simulink model "MCU_vectorControl_dsPIC33AK128MC106_MCLV_48V_300W"  (R2024a)
settings: Solver=FixedStepDiscrete  StartTime=0.0  StopTime=10.0  FixedStep=50e-6  RelTol=1e-3  EnableMultiTasking=on
undefined symbols (not defined in the file or in its folder): A0, A4, ADC, B0, Bias1, Bias2, C10, C11, C6, C7, C8, control, D11, D12, DiscIntNeverNeededParam, inverter, Max, MaxPer, model, ms, NumBits1, NumBits2, P1, P17, P20, P39, P40, P41, P43, P44, P60, P61, Pin, PosRange1, PosRange2, PWM1_Trg1, Resol, s, Slope1, Slope2, us
libraries: simulink x43, MCHP_Blockset x23
(part 5 of 5)

== system MCU_vectorControl_dsPIC33AK128MC106_MCLV_48V_300W/BOARD MCLV-48V-300W dsPIC33AK128MC106 MC DIM/Downsample x20 ==
  note: DownSample & Average by changing data scaling
  In1 : Inport
  Compare To Constant : simulink/Logic and Bit Operations/Compare To Constant  relop===  const=1  OutDataTypeStr=boolean
  Counter Limited : simulink/Sources/Counter Limited  uplimit=DownSample-1  tsamp=-1
  Data Type Duplicate : DataTypeDuplicate
  Data Type Propagation : simulink/Signal Attributes/Data Type Propagation  PropDataType=fixdt(1, 16)  IfRefDouble=double  IfRefSingle=single  IsSigned=IsSigned1 or IsSigned2  NumBitsBase=NumBits1+NumBits2  NumBitsMult=1  NumBitsAdd=0  NumBitsAllowFinal=1:128  PropScaling=2^-10  ValuesUsedBestPrec=[5 -7]  SlopeBase=Slope1  SlopeMult=1  SlopeAdd=0  BiasBase=Bias1  BiasMult=1  BiasAdd=0
  Data Type Propagation1 : simulink/Signal Attributes/Data Type Propagation  PropDataType=fixdt(1, 16)  IfRefDouble=double  IfRefSingle=single  IsSigned=IsSigned1 or IsSigned2  NumBitsBase=NumBits1+NumBits2  NumBitsMult=1  NumBitsAdd=0  NumBitsAllowFinal=1:128  PropScaling=2^-10  ValuesUsedBestPrec=[5 -7]  SlopeBase=PosRange1  SlopeMult=1  SlopeAdd=0  BiasBase=Bias1  BiasMult=1  BiasAdd=0
  Discrete-Time Integrator : DiscreteIntegrator  IntegratorMethod=Accumulation: Backward Euler  gainval=1  ExternalReset=sampled level  SampleTime=-1  OutDataTypeStr=Inherit: Inherit via back propagation  ICPrevOutput=DiscIntNeverNeededParam  ICPrevScaledInput=DiscIntNeverNeededParam
  Gain : Gain  Gain=1/DownSample  OutDataTypeStr=Inherit: Inherit via back propagation  RndMeth=Round
  Gain1 : Gain  Gain=1/DownSample  OutDataTypeStr=Inherit: Inherit via back propagation
  Rate Transition1 : RateTransition  OutPortSampleTimeOpt=Multiple of input port sample time  OutPortSampleTimeMultiple=DownSample  OutPortSampleTime=DownSample
  Rate Transition3 : RateTransition  OutPortSampleTimeOpt=Multiple of input port sample time  OutPortSampleTimeMultiple=DownSample  OutPortSampleTime=DownSample
  Terminator : Terminator
  Out1 : Outport  VectorParamsAs1DForOutWhenUnconnected=off
  wires:
  Gain1/1 -> Data Type Propagation1/3, Terminator/1
  Rate Transition1/1 -> Data Type Duplicate/1, Data Type Propagation1/1, Data Type Propagation1/2
  Gain/1 -> Out1/1, Data Type Duplicate/2
  Counter Limited/1 -> Compare To Constant/1
  Discrete-Time Integrator/1 -> Rate Transition3/1, Data Type Propagation/3
  Compare To Constant/1 -> Discrete-Time Integrator/2
  In1/1 -> Data Type Propagation/1, Data Type Propagation/2, Discrete-Time Integrator/1, Rate Transition1/1
  Rate Transition3/1 -> Gain/1, Gain1/1

== system MCU_vectorControl_dsPIC33AK128MC106_MCLV_48V_300W/BOARD MCLV-48V-300W dsPIC33AK128MC106 MC DIM/Downsample x20 _ ==
  note: DownSample & Average by changing data scaling
  In1 : Inport
  Compare To Constant : simulink/Logic and Bit Operations/Compare To Constant  relop===  const=1  OutDataTypeStr=boolean
  Counter Limited : simulink/Sources/Counter Limited  uplimit=DownSample-1  tsamp=-1
  Data Type Duplicate : DataTypeDuplicate
  Data Type Propagation : simulink/Signal Attributes/Data Type Propagation  PropDataType=fixdt(1, 16)  IfRefDouble=double  IfRefSingle=single  IsSigned=IsSigned1 or IsSigned2  NumBitsBase=NumBits1+NumBits2  NumBitsMult=1  NumBitsAdd=0  NumBitsAllowFinal=1:128  PropScaling=2^-10  ValuesUsedBestPrec=[5 -7]  SlopeBase=Slope1  SlopeMult=1  SlopeAdd=0  BiasBase=Bias1  BiasMult=1  BiasAdd=0
  Data Type Propagation1 : simulink/Signal Attributes/Data Type Propagation  PropDataType=fixdt(1, 16)  IfRefDouble=double  IfRefSingle=single  IsSigned=IsSigned1 or IsSigned2  NumBitsBase=NumBits1+NumBits2  NumBitsMult=1  NumBitsAdd=0  NumBitsAllowFinal=1:128  PropScaling=2^-10  ValuesUsedBestPrec=[5 -7]  SlopeBase=PosRange1  SlopeMult=1  SlopeAdd=0  BiasBase=Bias1  BiasMult=1  BiasAdd=0
  Discrete-Time Integrator : DiscreteIntegrator  IntegratorMethod=Accumulation: Backward Euler  gainval=1  ExternalReset=sampled level  SampleTime=-1  OutDataTypeStr=Inherit: Inherit via back propagation  ICPrevOutput=DiscIntNeverNeededParam  ICPrevScaledInput=DiscIntNeverNeededParam
  Gain : Gain  Gain=1/DownSample  OutDataTypeStr=Inherit: Inherit via back propagation  RndMeth=Round
  Gain1 : Gain  Gain=1/DownSample  OutDataTypeStr=Inherit: Inherit via back propagation
  Rate Transition1 : RateTransition  OutPortSampleTimeOpt=Multiple of input port sample time  OutPortSampleTimeMultiple=DownSample  OutPortSampleTime=DownSample
  Rate Transition3 : RateTransition  OutPortSampleTimeOpt=Multiple of input port sample time  OutPortSampleTimeMultiple=DownSample  OutPortSampleTime=DownSample
  Terminator : Terminator
  Out1 : Outport  VectorParamsAs1DForOutWhenUnconnected=off
  wires:
  Rate Transition3/1 -> Gain1/1, Gain/1
  In1/1 -> Rate Transition1/1, Discrete-Time Integrator/1, Data Type Propagation/2, Data Type Propagation/1
  Compare To Constant/1 -> Discrete-Time Integrator/2
  Discrete-Time Integrator/1 -> Data Type Propagation/3, Rate Transition3/1
  Counter Limited/1 -> Compare To Constant/1
  Gain/1 -> Data Type Duplicate/2, Out1/1
  Rate Transition1/1 -> Data Type Propagation1/2, Data Type Propagation1/1, Data Type Duplicate/1
  Gain1/1 -> Terminator/1, Data Type Propagation1/3

== system MCU_vectorControl_dsPIC33AK128MC106_MCLV_48V_300W/BOARD MCLV-48V-300W dsPIC33AK128MC106 MC DIM/MCLV 48V-300W board webpage ==

== system MCU_vectorControl_dsPIC33AK128MC106_MCLV_48V_300W/BOARD MCLV-48V-300W dsPIC33AK128MC106 MC DIM/Timing Analysis ==
  note: CPU overload is 0 if no overload took place between two MCU Overload block execution.
      | Otherwise, bits field output code for TID(s) responsible for at least one overload.
  Downsample Averaged2 : Subsystem  mask{InputSampleTime=.001, DownSample=100}
      mask prompts: InputSampleTime "Input sample time"; DownSample "DownSample Factor"
  Gain : Gain  Gain=5e-9/.001 * 100  OutMin=0  OutMax=100  OutDataTypeStr=fixdt(0,16)  RndMeth=Simplest  SaturateOnIntegerOverflow=on
  MCU Load : MCHP_Blockset/Profiling/MCU Load  MCULoadPin_TXT=None  MCULoadMeasure=on  TIMER_Resolution_TXT="Resol: 0.005(us)  -  Max: 0.328(ms)"  MCHP_TIMER_REQUEST={MCU_Load}{MCU_Load}21:5:0:0:[]:32768;  MCHP_TIMER_RESULT=[2 65535 ]  MCHP_MASTERLINK=MCU_vectorControl_dsPIC33AK128MC106_MCLV_48V_300W/BOARD MCLV-48V-300W dsPIC33AK128MC106 MC DIM/Microchip Master  MCHP_COMPILED_INFO="CompiledSampleTime= [0.0010000000000000000208   0 ];CompiledInportDataTypes=[    ];CompiledInportDataWidth=[];"  Info="Timer 2:  Resol: 5(ns)  -  Max: 327.68(us)"  SampleTime=.001
      settings: SourceProductName=MPLAB Device Blocks for Simulink
  MCU Overload : MCHP_Blockset/Profiling/MCU Overload  MCUOverloadBlockOutput=on  MCUOverLoadPin_TXT=None  MCHP_MASTERLINK=MCU_vectorControl_dsPIC33AK128MC106_MCLV_48V_300W/BOARD MCLV-48V-300W dsPIC33AK128MC106 MC DIM/Microchip Master  SampleTime=-1
      settings: SourceProductName=MPLAB Device Blocks for Simulink
  Overload : Constant  Value=65535  OutDataTypeStr=Inherit: Inherit via back propagation
  Rate Transition : RateTransition  Deterministic=off  OutPortSampleTime=.0005*200
  Switch : Switch  Criteria=u2 ~= 0  SaturateOnIntegerOverflow=off  InputSameDT=off
  CPU Load : Outport  Unit=%  SampleTime=.0005*200
  CPU Overload : Outport  Port=2
  wires:
  Gain/1 -> CPU Load/1
  Overload/1 -> Switch/1
  Switch/1 -> Gain/1
  Downsample Averaged2/1(Out1) -> Switch/3
  MCU Load/1 -> Downsample Averaged2/1(In1)
  MCU Overload/1 -> CPU Overload/1, Rate Transition/1
  Rate Transition/1 -> Switch/2

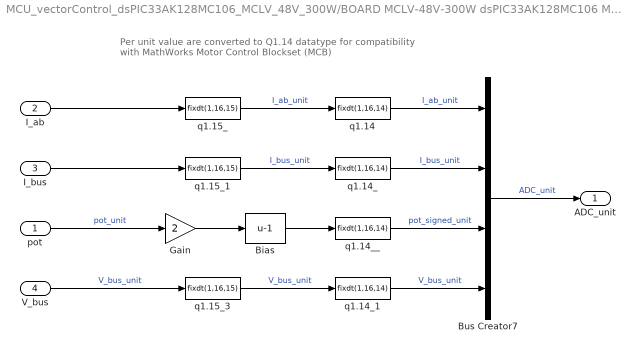
== system MCU_vectorControl_dsPIC33AK128MC106_MCLV_48V_300W/BOARD MCLV-48V-300W dsPIC33AK128MC106 MC DIM/per_unit ==
  note: Per unit value are converted to Q1.14 datatype
      | for compatibility with MathWorks Motor Control Blockset (MCB)
  pot : Inport
  I_ab : Inport  Port=2
  I_bus : Inport  Port=3
  V_bus : Inport  Port=4
  Bias : Bias  Bias=-1  SaturateOnIntegerOverflow=off
  Bus Creator7 : BusCreator  Inputs=4
  Gain : Gain  Gain=2  OutDataTypeStr=fixdt(1,16,15)  LockScale=on
  q1.14 : DataTypeConversion  OutDataTypeStr=fixdt(1,16,14)  SaturateOnIntegerOverflow=off  RndMeth=Floor  LockScale=on
  q1.14_ : DataTypeConversion  OutDataTypeStr=fixdt(1,16,14)  SaturateOnIntegerOverflow=off  RndMeth=Floor  LockScale=on
  q1.14_1 : DataTypeConversion  OutDataTypeStr=fixdt(1,16,14)  SaturateOnIntegerOverflow=off  RndMeth=Floor  LockScale=on
  q1.14__ : DataTypeConversion  OutDataTypeStr=fixdt(1,16,14)  SaturateOnIntegerOverflow=off  RndMeth=Floor  LockScale=on
  q1.15_ : DataTypeConversion  OutDataTypeStr=fixdt(1,16,15)  ConvertRealWorld=Stored Integer (SI)  SaturateOnIntegerOverflow=off  RndMeth=Floor  LockScale=on
  q1.15_1 : DataTypeConversion  OutDataTypeStr=fixdt(1,16,15)  ConvertRealWorld=Stored Integer (SI)  SaturateOnIntegerOverflow=off  RndMeth=Floor  LockScale=on
  q1.15_3 : DataTypeConversion  OutDataTypeStr=fixdt(1,16,15)  ConvertRealWorld=Stored Integer (SI)  SaturateOnIntegerOverflow=off  RndMeth=Floor  LockScale=on
  ADC_unit : Outport
  wires:
  Bias/1 -> q1.14__/1
  Gain/1 -> Bias/1
  q1.14_1/1 -> Bus Creator7/4  "V_bus_unit"
  q1.14__/1 -> Bus Creator7/3  "pot_signed_unit"
  q1.14_/1 -> Bus Creator7/2  "I_bus_unit"
  q1.14/1 -> Bus Creator7/1  "I_ab_unit"
  q1.15_3/1 -> q1.14_1/1  "V_bus_unit"
  Bus Creator7/1 -> ADC_unit/1  "ADC_unit"
  q1.15_/1 -> q1.14/1  "I_ab_unit"
  q1.15_1/1 -> q1.14_/1  "I_bus_unit"
  I_bus/1 -> q1.15_1/1
  pot/1 -> Gain/1  "pot_unit"
  V_bus/1 -> q1.15_3/1  "V_bus_unit"
  I_ab/1 -> q1.15_/1

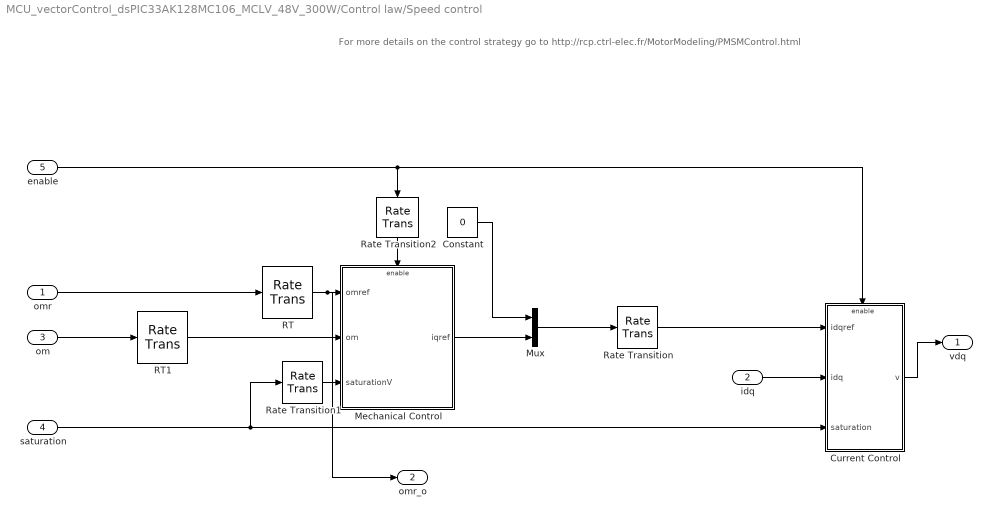
== system MCU_vectorControl_dsPIC33AK128MC106_MCLV_48V_300W/Control law/Speed control ==
  note: For more details on the control strategy go to
      |
      | http://rcp.ctrl-elec.fr/MotorModeling/PMSMControl.html
  omr : Inport
  idq : Inport  Port=2
  om : Inport  Port=3
  saturation : Inport  Port=4
  enable : Inport  Port=5
  Constant : Constant  Value=0  OutDataTypeStr=Inherit: Inherit via back propagation
  Current Control : Subsystem
  Mechanical Control : Subsystem
  Mux : Mux  Inputs=2
  RT : RateTransition  OutPortSampleTime=0.001
  RT1 : RateTransition  OutPortSampleTime=0.001
  Rate Transition : RateTransition
  Rate Transition1 : RateTransition  OutPortSampleTime=control.tsMeca
  Rate Transition2 : RateTransition
  vdq : Outport
  omr_o : Outport  Port=2
  wires:
  RT1/1 -> Mechanical Control/2(om)
  RT/1 -> omr_o/1, Mechanical Control/1(omref)
  idq/1 -> Current Control/2(idq)
  Mux/1 -> Rate Transition/1
  Current Control/1(v) -> vdq/1
  saturation/1 -> Rate Transition1/1, Current Control/3(saturation)
  om/1 -> RT1/1
  Constant/1 -> Mux/1
  Mechanical Control/1(iqref) -> Mux/2
  Rate Transition/1 -> Current Control/1(idqref)
  omr/1 -> RT/1
  Rate Transition1/1 -> Mechanical Control/3(saturationV)
  enable/1 -> Current Control/Enable, Rate Transition2/1
  Rate Transition2/1 -> Mechanical Control/Enable

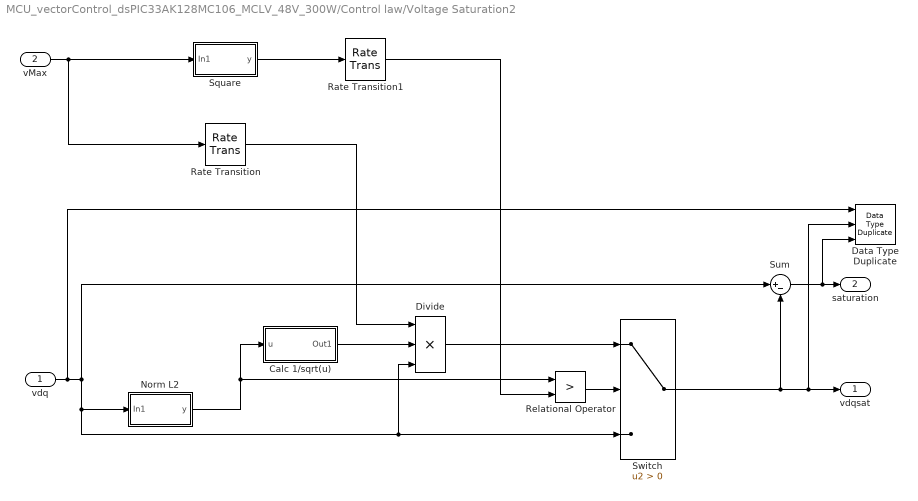
== system MCU_vectorControl_dsPIC33AK128MC106_MCLV_48V_300W/Control law/Voltage Saturation2 ==
  vdq : Inport
  vMax : Inport  Port=2
  Calc 1/sqrt(u) : Subsystem
  Data Type Duplicate : DataTypeDuplicate  NumInputPorts=3
  Divide : Product  Inputs=***  OutDataTypeStr=Inherit: Inherit via back propagation  SaturateOnIntegerOverflow=on
  Norm L2 : Subsystem
  Rate Transition : RateTransition
  Rate Transition1 : RateTransition
  Relational Operator : RelationalOperator  Operator=>  OutDataTypeStr=boolean  RndMeth=Simplest  InputSameDT=off
  Square : Subsystem
  Sum : Sum  Inputs=|+-  OutDataTypeStr=Inherit: Inherit via back propagation  SaturateOnIntegerOverflow=on
  Switch : Switch  Criteria=u2 > Threshold  OutDataTypeStr=Inherit: Inherit via back propagation  SaturateOnIntegerOverflow=off  InputSameDT=off
  vdqsat : Outport  VectorParamsAs1DForOutWhenUnconnected=off
  saturation : Outport  Port=2  VectorParamsAs1DForOutWhenUnconnected=off
  wires:
  Divide/1 -> Switch/1
  Norm L2/1(y) -> Calc 1/sqrt(u)/1(u), Relational Operator/1
  Switch/1 -> vdqsat/1, Data Type Duplicate/2, Sum/2
  vdq/1 -> Sum/1, Switch/3, Divide/3, Norm L2/1(In1), Data Type Duplicate/1
  Sum/1 -> saturation/1, Data Type Duplicate/3
  Relational Operator/1 -> Switch/2
  vMax/1 -> Square/1(In1), Rate Transition/1
  Square/1(y) -> Rate Transition1/1
  Rate Transition/1 -> Divide/1
  Rate Transition1/1 -> Relational Operator/2
  Calc 1/sqrt(u)/1(Out1) -> Divide/2

== system MCU_vectorControl_dsPIC33AK128MC106_MCLV_48V_300W/Control law/off1 ==
  Mux : Mux  Inputs=2
  vd : Constant  Value=0  OutDataTypeStr=Inherit: Inherit via back propagation
  vq : Constant  Value=0  OutDataTypeStr=Inherit: Inherit via back propagation
  vdq : Outport  VectorParamsAs1DForOutWhenUnconnected=off
  wires:
  vd/1 -> Mux/1
  Mux/1 -> vdq/1
  vq/1 -> Mux/2

== system MCU_vectorControl_dsPIC33AK128MC106_MCLV_48V_300W/Control law/open loop ==
  vdqr : Inport
  Enable : EnablePort
  vdq : Outport  VectorParamsAs1DForOutWhenUnconnected=off
  wires:
  vdqr/1 -> vdq/1

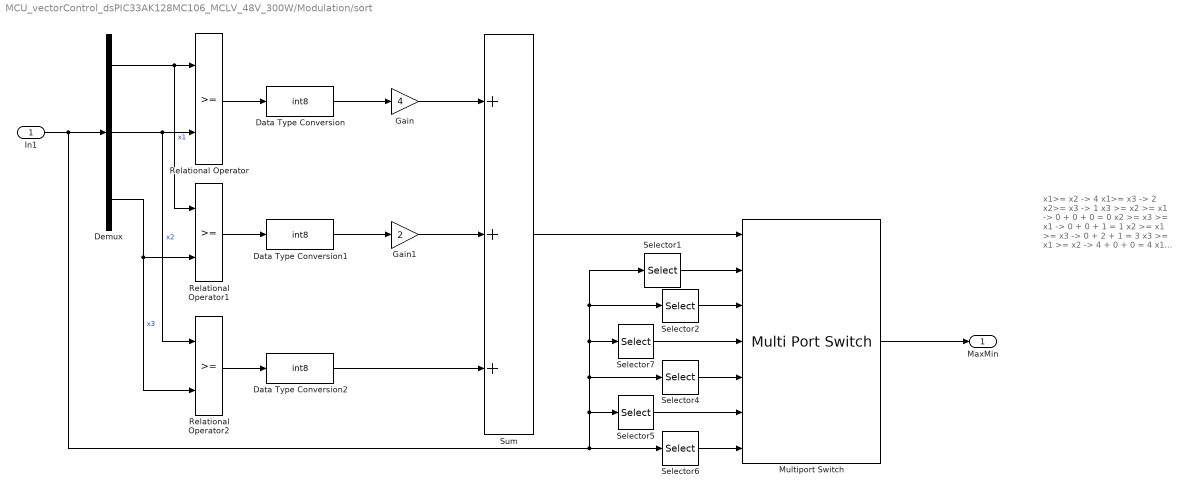
== system MCU_vectorControl_dsPIC33AK128MC106_MCLV_48V_300W/Modulation/sort ==
  note: x1>= x2 -> 4
      | x1>= x3 -> 2
      | x2>= x3 -> 1
      |
      | x3 >= x2 >= x1 -> 0 + 0 + 0 = 0
      | x2 >= x3 >= x1 -> 0 + 0 + 1 = 1
      | x2 >= x1 >= x3 -> 0 + 2 + 1 = 3
      | x3 >= x1 >= x2 -> 4 + 0 + 0 = 4
      | x1 >= x3 >= x2 -> 4 + 2 + 0 = 6
      | x1 >= x2 >= x3 -> 4 + 2 + 1 = 7
  In1 : Inport
  Data Type Conversion : DataTypeConversion  OutDataTypeStr=int8  SaturateOnIntegerOverflow=off  RndMeth=Floor
  Data Type Conversion1 : DataTypeConversion  OutDataTypeStr=int8  SaturateOnIntegerOverflow=off  RndMeth=Floor
  Data Type Conversion2 : DataTypeConversion  OutDataTypeStr=int8  SaturateOnIntegerOverflow=off  RndMeth=Floor
  Demux : Demux  Outputs=3
  Gain : Gain  Gain=4  OutDataTypeStr=Inherit: Same as input
  Gain1 : Gain  Gain=2  OutDataTypeStr=Inherit: Same as input
  Multiport Switch : MultiPortSwitch  DataPortOrder=Specify indices  DataPortIndices={0,1,3,4,6,7}  SaturateOnIntegerOverflow=off  InputSameDT=off
  Relational Operator : RelationalOperator  OutDataTypeStr=boolean  RndMeth=Simplest  InputSameDT=off
  Relational Operator1 : RelationalOperator  OutDataTypeStr=boolean  RndMeth=Simplest  InputSameDT=off
  Relational Operator2 : RelationalOperator  OutDataTypeStr=boolean  RndMeth=Simplest  InputSameDT=off
  Selector1 : Selector  InputPortWidth=3  IndexOptions=Index vector (dialog)  Indices=[3 1]  OutputSizes=1
  Selector2 : Selector  InputPortWidth=3  IndexOptions=Index vector (dialog)  Indices=[2 1]  OutputSizes=1
  Selector4 : Selector  InputPortWidth=3  IndexOptions=Index vector (dialog)  Indices=[3 2]  OutputSizes=1
  Selector5 : Selector  InputPortWidth=3  IndexOptions=Index vector (dialog)  Indices=[1 2]  OutputSizes=1
  Selector6 : Selector  InputPortWidth=3  IndexOptions=Index vector (dialog)  Indices=[1 3]  OutputSizes=1
  Selector7 : Selector  InputPortWidth=3  IndexOptions=Index vector (dialog)  Indices=[2 3]  OutputSizes=1
  Sum : Sum  Inputs=+++
  MaxMin : Outport
  wires:
  Demux/3 -> Relational Operator2/2, Relational Operator1/2  "x3"
  Demux/2 -> Relational Operator2/1, Relational Operator/2  "x2"
  Demux/1 -> Relational Operator1/1, Relational Operator/1  "x1"
  In1/1 -> Selector4/1, Selector7/1, Selector2/1, Selector1/1, Selector5/1, Selector6/1, Demux/1
  Relational Operator2/1 -> Data Type Conversion2/1
  Relational Operator1/1 -> Data Type Conversion1/1
  Relational Operator/1 -> Data Type Conversion/1
  Data Type Conversion/1 -> Gain/1
  Data Type Conversion1/1 -> Gain1/1
  Gain1/1 -> Sum/2
  Gain/1 -> Sum/1
  Data Type Conversion2/1 -> Sum/3
  Sum/1 -> Multiport Switch/1
  Selector1/1 -> Multiport Switch/2
  Selector6/1 -> Multiport Switch/7
  Selector5/1 -> Multiport Switch/6
  Selector4/1 -> Multiport Switch/5
  Selector7/1 -> Multiport Switch/4
  Selector2/1 -> Multiport Switch/3
  Multiport Switch/1 -> MaxMin/1

== system MCU_vectorControl_dsPIC33AK128MC106_MCLV_48V_300W/Park/Clarke ==
  note: Clark transform
      | $x_{\alpha\beta} = \frac{2}{3}\underbrace{\left[\begin{array}{ccc}1&-\frac{1}{2}&-\frac{1}{2}\\0&\frac{\sqrt{3}}{2}&-\frac{\sqrt{3}}{2}\end{array}\right]}_{C_{23}}x_{abc}$
      | if only 2 currents are measured since $x_a+x_b+x_c = 0$
      | $x_{abc} = \left[\begin{array}{cc}1 & 0\\0 & 1\\-1&-1\end{array}\right]x_{ab}$
      | leading to
      | $x_{\alpha\beta} = \underbrace{\left[\begin{array}{cc}1&0\\\frac{1}{\sqrt{3}}&\frac{2}{\sqrt{3}}\end{array}\right]}_{C_{22}}x_{ab}$
  xab(c) : Inport
  C1 : Gain  Gain=[1/sqrt(3) 2/sqrt(3)]  Multiplication=Matrix(K*u)  OutDataTypeStr=Inherit: Same as input
  Mux : Mux  Inputs=2
  Selector : Selector  InputPortWidth=2  IndexOptions=Index vector (dialog)  Indices=[1]  OutputSizes=1
  xalphabeta : Outport  VectorParamsAs1DForOutWhenUnconnected=off
  wires:
  xab(c)/1 -> Selector/1, C1/1
  Mux/1 -> xalphabeta/1
  Selector/1 -> Mux/1
  C1/1 -> Mux/2

== system MCU_vectorControl_dsPIC33AK128MC106_MCLV_48V_300W/Park/Park ==
  note: Park
      | $x_{dq} = P(\theta)^{-1}x_{\alpha\beta}\\ P(p\theta)^{-1} = \left[\begin{array}{cc}\cos(p\theta) & \sin(p\theta)\\ -\sin(p\theta) & \cos(p\theta) \end{array}\right]$
  xalphabeta : Inport  PortDimensions=2
  P(pth) : Inport  Port=2
  Data Type Duplicate2 : DataTypeDuplicate
  Park : Product  Multiplication=Matrix(*)  OutDataTypeStr=Inherit: Inherit via back propagation  RndMeth=Round
  xdq : Outport  VectorParamsAs1DForOutWhenUnconnected=off
  wires:
  Park/1 -> Data Type Duplicate2/1, xdq/1
  xalphabeta/1 -> Data Type Duplicate2/2, Park/2
  P(pth)/1 -> Park/1

== system MCU_vectorControl_dsPIC33AK128MC106_MCLV_48V_300W/Park inverse/Clarke Inverse ==
  note: Clarke inverse
  xalphabeta : Inport
  C23' : Gain  Gain=|  Multiplication=Matrix(K*u)  OutDataTypeStr=Inherit: Inherit via back propagation  RndMeth=Round
      | [1   -1/2        -1/2;
      |         0   sqrt(3)/2   -sqrt(3)/2]'
  xabc : Outport  VectorParamsAs1DForOutWhenUnconnected=off
  wires:
  C23'/1 -> xabc/1
  xalphabeta/1 -> C23'/1

== system MCU_vectorControl_dsPIC33AK128MC106_MCLV_48V_300W/Park inverse/Park inverse ==
  note: Inverse Park
      | $x_{\alpha\beta} = P(p\theta)x_{dq}\\ P(p\theta) = \left[\begin{array}{cc}\cos(p\theta) & -\sin(p\theta)\\ \sin(p\theta) & \cos(p\theta) \end{array}\right]$
  xdq : Inport
  P(pth) : Inport  Port=2
  Data Type Duplicate2 : DataTypeDuplicate
  Transpose : Math  Operator=transpose
  Transpose1 : Math  Operator=transpose
  xalpha sin(pth)1 : Product  Multiplication=Matrix(*)  OutDataTypeStr=Inherit: Inherit via back propagation  RndMeth=Round
  xalpahbeta : Outport  VectorParamsAs1DForOutWhenUnconnected=off
  wires:
  xalpha sin(pth)1/1 -> Transpose1/1, Data Type Duplicate2/1
  xdq/1 -> Transpose/1
  Transpose/1 -> xalpha sin(pth)1/1, Data Type Duplicate2/2
  Transpose1/1 -> xalpahbeta/1
  P(pth)/1 -> xalpha sin(pth)1/2

== system MCU_vectorControl_dsPIC33AK128MC106_MCLV_48V_300W/Referances Selector/Direction Toggle ==
  in : Inport
  Change when button is pressed : simulink/Logic and Bit Operations/Detect Decrease  vinit=0.0  OutDataTypeStr=uint8
  Logical Operator : Logic  Operator=XOR  AllPortsSameDT=off  OutDataTypeStr=boolean
  Unit Delay : UnitDelay  SampleTime=-1  HasFrameUpgradeWarning=on
  Toggle : Outport  VectorParamsAs1DForOutWhenUnconnected=off
  wires:
  Unit Delay/1 -> Logical Operator/2
  Change when button is pressed/1 -> Logical Operator/1
  in/1 -> Change when button is pressed/1
  Logical Operator/1 -> Toggle/1, Unit Delay/1  "Toggle"

== system MCU_vectorControl_dsPIC33AK128MC106_MCLV_48V_300W/Referances Selector/Direction Toggle1 ==
  in : Inport
  Change when button is pressed : simulink/Logic and Bit Operations/Detect Decrease  vinit=0.0  OutDataTypeStr=uint8
  Logical Operator : Logic  Operator=XOR  AllPortsSameDT=off  OutDataTypeStr=boolean
  Unit Delay : UnitDelay  SampleTime=-1  HasFrameUpgradeWarning=on
  Toggle : Outport  VectorParamsAs1DForOutWhenUnconnected=off
  wires:
  Logical Operator/1 -> Unit Delay/1, Toggle/1  "Toggle"
  in/1 -> Change when button is pressed/1
  Change when button is pressed/1 -> Logical Operator/1
  Unit Delay/1 -> Logical Operator/2

== system MCU_vectorControl_dsPIC33AK128MC106_MCLV_48V_300W/Referances Selector/Mode Toggle ==
  state : Inport
  Change when button is pressed : simulink/Logic and Bit Operations/Detect Decrease  vinit=0.0  OutDataTypeStr=uint8
  Compare To Constant : simulink/Logic and Bit Operations/Compare To Constant  relop=>  const=5  OutDataTypeStr=boolean
  Delay : Delay  DelayLength=1
  Discrete-Time Integrator : DiscreteIntegrator  IntegratorMethod=Accumulation: Forward Euler  ExternalReset=sampled level  SampleTime=-1  ICPrevOutput=DiscIntNeverNeededParam  ICPrevScaledInput=DiscIntNeverNeededParam
  Mode : Outport  PortDimensions=1  VectorParamsAs1DForOutWhenUnconnected=off
  wires:
  state/1 -> Change when button is pressed/1
  Delay/1 -> Compare To Constant/1
  Discrete-Time Integrator/1 -> Mode/1, Delay/1
  Change when button is pressed/1 -> Discrete-Time Integrator/1
  Compare To Constant/1 -> Discrete-Time Integrator/2

== system MCU_vectorControl_dsPIC33AK128MC106_MCLV_48V_300W/BOARD MCLV-48V-300W dsPIC33AK128MC106 MC DIM/Center & sign reversal/Downsample Averaged 2000 samples remove bias ==
  note: DownSample & Average by changing data scaling
  In1 : Inport
  Enable : EnablePort
  Compare To Constant : simulink/Logic and Bit Operations/Compare To Constant  relop===  const=1  OutDataTypeStr=boolean
  Counter Limited : simulink/Sources/Counter Limited  uplimit=DownSample-1  tsamp=-1
  Data Type Duplicate : DataTypeDuplicate
  Data Type Propagation : simulink/Signal Attributes/Data Type Propagation  PropDataType=fixdt(1, 16)  IfRefDouble=double  IfRefSingle=single  IsSigned=IsSigned1 or IsSigned2  NumBitsBase=NumBits1+NumBits2  NumBitsMult=1  NumBitsAdd=0  NumBitsAllowFinal=1:128  PropScaling=2^-10  ValuesUsedBestPrec=[5 -7]  SlopeBase=Slope1  SlopeMult=1  SlopeAdd=0  BiasBase=Bias1  BiasMult=1  BiasAdd=0
  Data Type Propagation1 : simulink/Signal Attributes/Data Type Propagation  PropDataType=fixdt(1, 16)  IfRefDouble=double  IfRefSingle=single  IsSigned=IsSigned1 or IsSigned2  NumBitsBase=NumBits1+NumBits2  NumBitsMult=1  NumBitsAdd=0  NumBitsAllowFinal=1:128  PropScaling=2^-10  ValuesUsedBestPrec=[5 -7]  SlopeBase=PosRange1  SlopeMult=1  SlopeAdd=0  BiasBase=Bias1  BiasMult=1  BiasAdd=0
  Discrete-Time Integrator : DiscreteIntegrator  IntegratorMethod=Accumulation: Backward Euler  gainval=1  ExternalReset=sampled level  SampleTime=-1  OutDataTypeStr=Inherit: Inherit via back propagation  ICPrevOutput=DiscIntNeverNeededParam  ICPrevScaledInput=DiscIntNeverNeededParam
  Gain : Gain  Gain=1/DownSample  OutDataTypeStr=Inherit: Inherit via back propagation  RndMeth=Round
  Gain1 : Gain  Gain=1/DownSample  OutDataTypeStr=Inherit: Inherit via back propagation
  Rate Transition1 : RateTransition  OutPortSampleTimeOpt=Multiple of input port sample time  OutPortSampleTimeMultiple=DownSample  OutPortSampleTime=DownSample
  Rate Transition3 : RateTransition  OutPortSampleTimeOpt=Multiple of input port sample time  OutPortSampleTimeMultiple=DownSample  OutPortSampleTime=DownSample
  Terminator : Terminator
  Out1 : Outport  InitialOutput=[32768]  VectorParamsAs1DForOutWhenUnconnected=off
  wires:
  Rate Transition3/1 -> Gain1/1, Gain/1
  In1/1 -> Rate Transition1/1, Discrete-Time Integrator/1, Data Type Propagation/2, Data Type Propagation/1
  Compare To Constant/1 -> Discrete-Time Integrator/2
  Discrete-Time Integrator/1 -> Data Type Propagation/3, Rate Transition3/1
  Counter Limited/1 -> Compare To Constant/1
  Gain/1 -> Data Type Duplicate/2, Terminator/1
  Rate Transition1/1 -> Data Type Propagation1/2, Data Type Propagation1/1, Data Type Duplicate/1
  Gain1/1 -> Data Type Propagation1/3, Out1/1

== system MCU_vectorControl_dsPIC33AK128MC106_MCLV_48V_300W/BOARD MCLV-48V-300W dsPIC33AK128MC106 MC DIM/Timing Analysis/Downsample Averaged2 ==
  note: DownSample & Average by changing data scaling
  In1 : Inport
  Compare To Constant : simulink/Logic and Bit Operations/Compare To Constant  relop===  const=1  OutDataTypeStr=boolean
  Counter Limited : simulink/Sources/Counter Limited  uplimit=DownSample-1  tsamp=-1
  Data Type Duplicate : DataTypeDuplicate
  Data Type Propagation : simulink/Signal Attributes/Data Type Propagation  PropDataType=fixdt(1, 16)  IfRefDouble=double  IfRefSingle=single  IsSigned=IsSigned1 or IsSigned2  NumBitsBase=NumBits1+NumBits2  NumBitsMult=1  NumBitsAdd=0  NumBitsAllowFinal=1:128  PropScaling=2^-10  ValuesUsedBestPrec=[5 -7]  SlopeBase=Slope1  SlopeMult=1  SlopeAdd=0  BiasBase=Bias1  BiasMult=1  BiasAdd=0
  Data Type Propagation1 : simulink/Signal Attributes/Data Type Propagation  PropDataType=fixdt(1, 16)  IfRefDouble=double  IfRefSingle=single  IsSigned=IsSigned1 or IsSigned2  NumBitsBase=NumBits1+NumBits2  NumBitsMult=1  NumBitsAdd=0  NumBitsAllowFinal=1:128  PropScaling=2^-10  ValuesUsedBestPrec=[5 -7]  SlopeBase=PosRange1  SlopeMult=1  SlopeAdd=0  BiasBase=Bias1  BiasMult=1  BiasAdd=0
  Discrete-Time Integrator : DiscreteIntegrator  IntegratorMethod=Accumulation: Backward Euler  gainval=1  ExternalReset=sampled level  SampleTime=-1  OutDataTypeStr=Inherit: Inherit via back propagation  ICPrevOutput=DiscIntNeverNeededParam  ICPrevScaledInput=DiscIntNeverNeededParam
  Gain : Gain  Gain=1/DownSample  OutDataTypeStr=Inherit: Inherit via back propagation
  Gain1 : Gain  Gain=1/DownSample  OutDataTypeStr=Inherit: Inherit via back propagation
  Rate Transition1 : RateTransition  Deterministic=off  OutPortSampleTime=[InputSampleTime * DownSample]
  Rate Transition3 : RateTransition  OutPortSampleTime=[InputSampleTime * DownSample]
  Terminator : Terminator
  Out1 : Outport  VectorParamsAs1DForOutWhenUnconnected=off
  wires:
  Gain1/1 -> Terminator/1, Data Type Propagation1/3
  Rate Transition1/1 -> Data Type Duplicate/1, Data Type Propagation1/1, Data Type Propagation1/2
  Gain/1 -> Out1/1, Data Type Duplicate/2
  Counter Limited/1 -> Compare To Constant/1
  Discrete-Time Integrator/1 -> Rate Transition3/1, Data Type Propagation/3
  Compare To Constant/1 -> Discrete-Time Integrator/2
  In1/1 -> Data Type Propagation/1, Data Type Propagation/2, Rate Transition1/1, Discrete-Time Integrator/1
  Rate Transition3/1 -> Gain/1, Gain1/1

== system MCU_vectorControl_dsPIC33AK128MC106_MCLV_48V_300W/Control law/Speed control/Current Control ==
  idqref : Inport
  idq : Inport  Port=2
  saturation : Inport  Port=3
  Enable : EnablePort  StatesWhenEnabling=reset
  Clamping circuit : Subsystem
  Data Type Conversion : DataTypeConversion  SaturateOnIntegerOverflow=off  RndMeth=Floor
  Discrete-Time Integrator : DiscreteIntegrator  SampleTime=-1  OutDataTypeStr=Inherit: Inherit via back propagation  SaturateOnIntegerOverflow=on  ICPrevOutput=DiscIntNeverNeededParam  ICPrevScaledInput=DiscIntNeverNeededParam
  Gain : Gain  Gain=control.kE(2)  OutDataTypeStr=Inherit: Inherit via back propagation  SaturateOnIntegerOverflow=on
  Gain1 : Gain  Gain=control.kE(1)  OutDataTypeStr=Inherit: Inherit via back propagation  SaturateOnIntegerOverflow=on
  Product : Product  OutDataTypeStr=Inherit: Same as first input
  Sum : Sum  Inputs=|--  OutDataTypeStr=Inherit: Inherit via back propagation  SaturateOnIntegerOverflow=on
  Sum3 : Sum  Inputs=|+-  OutDataTypeStr=Inherit: Inherit via back propagation  SaturateOnIntegerOverflow=on
  v : Outport  VectorParamsAs1DForOutWhenUnconnected=off
  wires:
  Sum3/1 -> Clamping circuit/1(preIntegrator), Gain/1
  Gain/1 -> Product/1
  Clamping circuit/1(Clamp) -> Product/2
  Product/1 -> Discrete-Time Integrator/1
  saturation/1 -> Clamping circuit/2(saturation)
  Gain1/1 -> Sum/2
  Discrete-Time Integrator/1 -> Data Type Conversion/1
  idq/1 -> Gain1/1, Sum3/2
  idqref/1 -> Sum3/1
  Sum/1 -> v/1
  Data Type Conversion/1 -> Sum/1

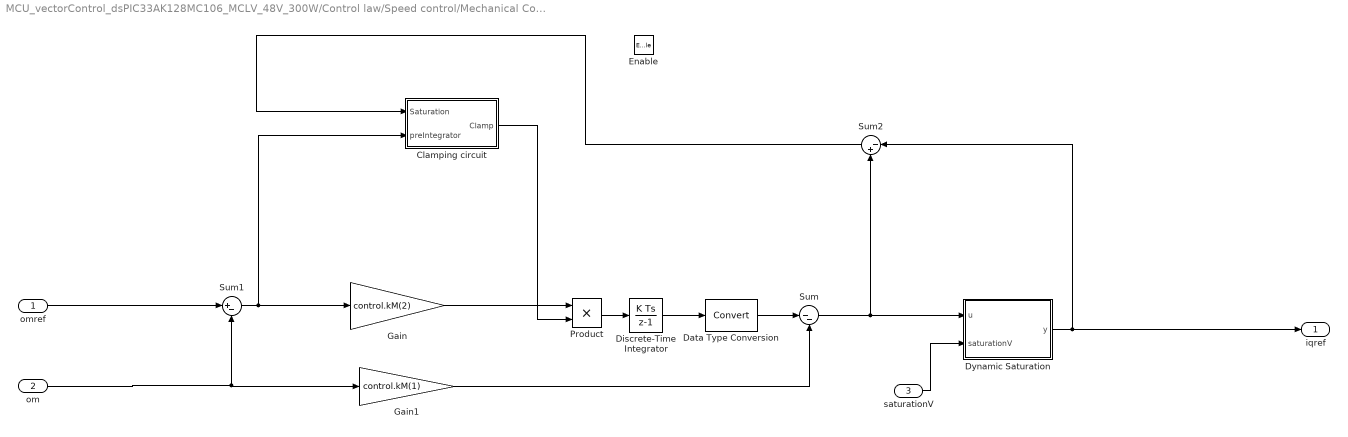
== system MCU_vectorControl_dsPIC33AK128MC106_MCLV_48V_300W/Control law/Speed control/Mechanical Control ==
  omref : Inport
  om : Inport  Port=2
  saturationV : Inport  Port=3
  Enable : EnablePort  StatesWhenEnabling=reset
  Clamping circuit : Subsystem
  Data Type Conversion : DataTypeConversion  SaturateOnIntegerOverflow=off  RndMeth=Floor
  Discrete-Time Integrator : DiscreteIntegrator  SampleTime=-1  OutDataTypeStr=Inherit: Inherit via back propagation  SaturateOnIntegerOverflow=on  ICPrevOutput=DiscIntNeverNeededParam  ICPrevScaledInput=DiscIntNeverNeededParam
  Dynamic Saturation : Subsystem
  Gain : Gain  Gain=control.kM(2)  OutDataTypeStr=Inherit: Inherit via back propagation  SaturateOnIntegerOverflow=on
  Gain1 : Gain  Gain=control.kM(1)  OutDataTypeStr=Inherit: Inherit via back propagation  SaturateOnIntegerOverflow=on
  Product : Product  OutDataTypeStr=Inherit: Same as first input
  Sum : Sum  Inputs=|--  OutDataTypeStr=Inherit: Inherit via back propagation  SaturateOnIntegerOverflow=on
  Sum1 : Sum  Inputs=|+-  OutDataTypeStr=Inherit: Inherit via back propagation
  Sum2 : Sum  Inputs=|-+  SaturateOnIntegerOverflow=on  OutDataTypeStr=Inherit: Same as first input
  iqref : Outport  VectorParamsAs1DForOutWhenUnconnected=off
  wires:
  Sum1/1 -> Clamping circuit/2(preIntegrator), Gain/1
  Gain/1 -> Product/1
  Product/1 -> Discrete-Time Integrator/1
  saturationV/1 -> Dynamic Saturation/2(saturationV)
  Gain1/1 -> Sum/2
  Sum2/1 -> Clamping circuit/1(Saturation)
  Clamping circuit/1(Clamp) -> Product/2
  omref/1 -> Sum1/1
  om/1 -> Gain1/1, Sum1/2
  Discrete-Time Integrator/1 -> Data Type Conversion/1
  Sum/1 -> Dynamic Saturation/1(u), Sum2/2
  Dynamic Saturation/1(y) -> iqref/1, Sum2/1
  Data Type Conversion/1 -> Sum/1

== system MCU_vectorControl_dsPIC33AK128MC106_MCLV_48V_300W/Control law/Voltage Saturation2/Calc 1//sqrt(u) ==
  u : Inport
  Reciprocal : Product  Inputs=/
  Sqrt : Sqrt
  Out1 : Outport
  wires:
  Sqrt/1 -> Reciprocal/1
  u/1 -> Sqrt/1
  Reciprocal/1 -> Out1/1

== system MCU_vectorControl_dsPIC33AK128MC106_MCLV_48V_300W/Control law/Voltage Saturation2/Norm L2 ==
  In1 : Inport
  Data Type Propagation : simulink/Signal Attributes/Data Type Propagation  PropDataType=fixdt(1, 16)  IfRefDouble=double  IfRefSingle=single  IsSigned=IsSigned1 or IsSigned2  NumBitsBase=max([NumBits1 NumBits2])  NumBitsMult=1  NumBitsAdd=0  NumBitsAllowFinal=1:128  PropScalingMode=Specify via dialog  PropScaling=2^-model.FracLen.volt2  ValuesUsedBestPrec=[5 -7]  SlopeBase=PosRange1*PosRange2  SlopeMult=1  SlopeAdd=0  BiasBase=max([Bias1 Bias2])  BiasMult=1  BiasAdd=0
  Dot Product : DotProduct  OutDataTypeStr=Inherit: Inherit via back propagation  SaturateOnIntegerOverflow=on
  y : Outport
  wires:
  Dot Product/1 -> y/1, Data Type Propagation/3
  In1/1 -> Dot Product/1, Dot Product/2, Data Type Propagation/2, Data Type Propagation/1

== system MCU_vectorControl_dsPIC33AK128MC106_MCLV_48V_300W/Control law/Voltage Saturation2/Square ==
  In1 : Inport
  Data Type Propagation : simulink/Signal Attributes/Data Type Propagation  PropDataType=fixdt(1, 16)  IfRefDouble=double  IfRefSingle=single  IsSigned=IsSigned1 or IsSigned2  NumBitsBase=max([NumBits1 NumBits2])  NumBitsMult=1  NumBitsAdd=0  NumBitsAllowFinal=1:128  PropScalingMode=Specify via dialog  PropScaling=2^-model.FracLen.volt2  ValuesUsedBestPrec=[5 -7]  SlopeBase=PosRange1*PosRange2  SlopeMult=1  SlopeAdd=0  BiasBase=max([Bias1 Bias2])  BiasMult=1  BiasAdd=0
  Square : Math  Operator=square  OutDataTypeStr=Inherit: Inherit via back propagation
  y : Outport
  wires:
  In1/1 -> Data Type Propagation/1, Data Type Propagation/2, Square/1
  Square/1 -> y/1, Data Type Propagation/3

== system MCU_vectorControl_dsPIC33AK128MC106_MCLV_48V_300W/Control law/Speed control/Current Control/Clamping circuit ==
  note: The clamping enable or disable the integral action.
  preIntegrator : Inport  DisableCoverage=on
  saturation : Inport  DisableCoverage=on  Port=2
  AND : Logic  Operator=OR  IconShape=distinctive  AllPortsSameDT=off  OutDataTypeStr=boolean
  Compare To Zero1 : simulink/Logic and Bit Operations/Compare To Zero  relop=<=  OutDataTypeStr=boolean
  Delay : Delay  DelayLength=1
  Demux : Demux  Outputs=2
  Multiply : Product
  Clamp : Outport  DisableCoverage=on  VectorParamsAs1DForOutWhenUnconnected=off
  wires:
  Delay/1 -> Multiply/1
  Demux/1 -> AND/1
  Demux/2 -> AND/2
  AND/1 -> Clamp/1
  preIntegrator/1 -> Multiply/2
  Multiply/1 -> Compare To Zero1/1
  Compare To Zero1/1 -> Demux/1
  saturation/1 -> Delay/1

== system MCU_vectorControl_dsPIC33AK128MC106_MCLV_48V_300W/Control law/Speed control/Mechanical Control/Clamping circuit ==
  note: The clamping enable or disable the integral action.
  Saturation : Inport  DisableCoverage=on
  preIntegrator : Inport  DisableCoverage=on  Port=2
  Compare To Zero1 : simulink/Logic and Bit Operations/Compare To Zero  relop=<=  OutDataTypeStr=boolean
  Delay : Delay  DelayLength=1  InitialCondition=0
  Multiply : Product
  Clamp : Outport  DisableCoverage=on  VectorParamsAs1DForOutWhenUnconnected=off
  wires:
  Compare To Zero1/1 -> Clamp/1
  preIntegrator/1 -> Multiply/2
  Multiply/1 -> Compare To Zero1/1
  Saturation/1 -> Delay/1
  Delay/1 -> Multiply/1

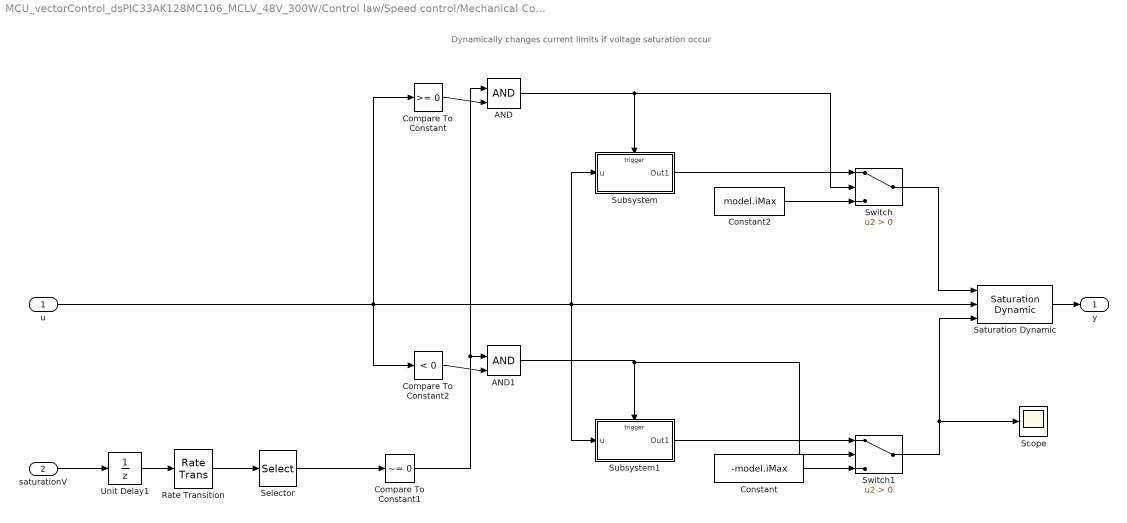
== system MCU_vectorControl_dsPIC33AK128MC106_MCLV_48V_300W/Control law/Speed control/Mechanical Control/Dynamic Saturation ==
  note: Dynamically changes current limits if voltage saturation occur
  u : Inport
  saturationV : Inport  Port=2
  AND : Logic  IconShape=distinctive  AllPortsSameDT=off  OutDataTypeStr=boolean
  AND1 : Logic  IconShape=distinctive  AllPortsSameDT=off  OutDataTypeStr=boolean
  Compare To Constant : simulink/Logic and Bit Operations/Compare To Constant  relop=>=  const=0  OutDataTypeStr=boolean
  Compare To Constant1 : simulink/Logic and Bit Operations/Compare To Constant  relop=~=  const=0  OutDataTypeStr=boolean
  Compare To Constant2 : simulink/Logic and Bit Operations/Compare To Constant  relop=<  const=0  OutDataTypeStr=boolean
  Constant : Constant  Value=-model.iMax  OutDataTypeStr=single  SampleTime=1e-3
  Constant2 : Constant  Value=model.iMax  OutDataTypeStr=single  SampleTime=1e-3
  Rate Transition : RateTransition  OutPortSampleTime=control.tsMeca
  Saturation Dynamic : simulink/Discontinuities/Saturation Dynamic  OutMin=[]  OutMax=[]  OutDataTypeStr=Inherit: Same as second input  OutDataType=fixdt(1, 16)  OutScaling=2^-10  DoSatur=off
  Scope : Scope
  Selector : Selector  InputPortWidth=2  IndexOptions=Index vector (dialog)  Indices=2  OutputSizes=1
  Subsystem : Subsystem
  Subsystem1 : Subsystem
  Switch : Switch  Criteria=u2 > Threshold  SaturateOnIntegerOverflow=off  InputSameDT=off
  Switch1 : Switch  Criteria=u2 > Threshold  SaturateOnIntegerOverflow=off  InputSameDT=off
  Unit Delay1 : UnitDelay  SampleTime=-1  HasFrameUpgradeWarning=on
  y : Outport
  wires:
  Selector/1 -> Compare To Constant1/1
  Compare To Constant/1 -> AND/2
  Unit Delay1/1 -> Rate Transition/1
  Rate Transition/1 -> Selector/1
  Constant/1 -> Switch1/3
  Switch1/1 -> Saturation Dynamic/3, Scope/1
  Subsystem1/1(Out1) -> Switch1/1
  AND1/1 -> Switch1/2, Subsystem1/Trigger
  Compare To Constant2/1 -> AND1/2
  Subsystem/1(Out1) -> Switch/1
  Constant2/1 -> Switch/3
  AND/1 -> Subsystem/Trigger, Switch/2
  Compare To Constant1/1 -> AND1/1, AND/1
  saturationV/1 -> Unit Delay1/1
  Saturation Dynamic/1 -> y/1
  u/1 -> Saturation Dynamic/2, Subsystem1/1(u), Subsystem/1(u), Compare To Constant2/1, Compare To Constant/1
  Switch/1 -> Saturation Dynamic/1

== system MCU_vectorControl_dsPIC33AK128MC106_MCLV_48V_300W/Control law/Speed control/Mechanical Control/Dynamic Saturation/Subsystem ==
  u : Inport
  Trigger : TriggerPort  VariantControl=(inherit)  PortDimensions=1
  Out1 : Outport
  wires:
  u/1 -> Out1/1

== system MCU_vectorControl_dsPIC33AK128MC106_MCLV_48V_300W/Control law/Speed control/Mechanical Control/Dynamic Saturation/Subsystem1 ==
  u : Inport
  Trigger : TriggerPort  VariantControl=(inherit)  PortDimensions=1
  Out1 : Outport
  wires:
  u/1 -> Out1/1
